simulink model "AMCLIB_FWSpeedLoop_BAM_F16"  (Simulink 8.3)
settings: Solver=ode45  StartTime=0.0  StopTime=10.0  RelTol=1e-3
undefined symbols (not defined in the file): f16IntegGainFW, f16IntegGainQ, f16PropGainFW, f16PropGainQ, f32RampDown, f32RampUp, s16IntegGainShiftFW, s16IntegGainShiftQ, s16PropGainShiftFW, s16PropGainShiftQ, u16NSamplesFW, u16NSamplesW
settings Model: Creator=nxa18952  LastModifiedBy=nxa18952
settings DataIOCC: SignalLoggingSaveFormat=Dataset
settings DebuggingCC: UnderspecifiedInitializationDetection=Simplified  StateNameClashWarn=none
settings GRTTargetCC: CombineOutputUpdateFcns=on  GRTInterface=off

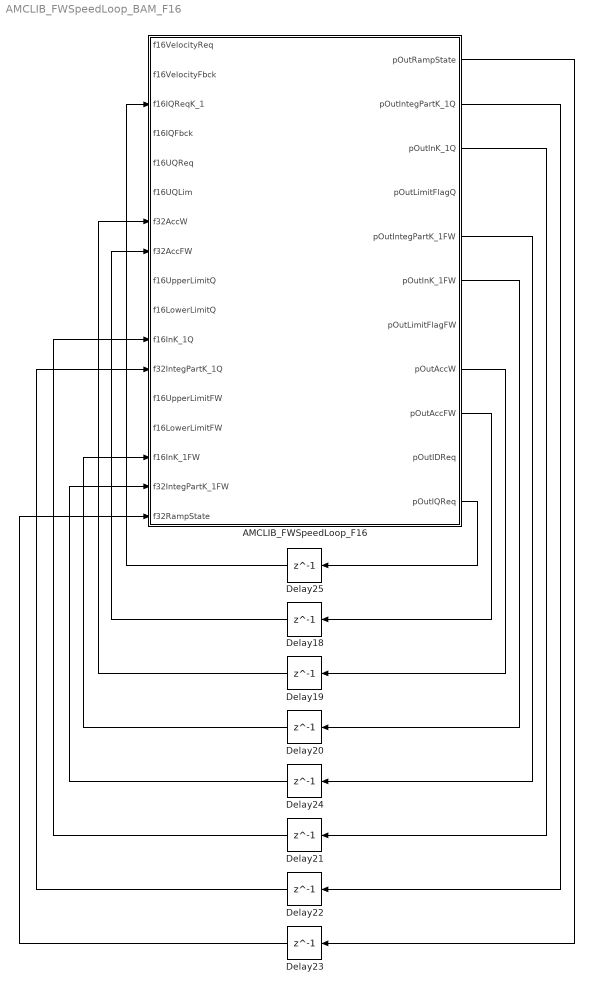
== system AMCLIB_FWSpeedLoop_BAM_F16 ==
  AMCLIB_FWSpeedLoop_F16 : Subsystem  mask(AMCLIB_FWSpeedLoop_F16){u16NSamplesW=u16NSamplesW, u16NSamplesFW=u16NSamplesFW, f16PropGainQ=f16PropGainQ, s16PropGainShiftQ=s16PropGainShiftQ, f16IntegGainQ=f16IntegGainQ, s16IntegGainShiftQ=s16IntegGainShiftQ, f16PropGainFW=f16PropGainFW, s16PropGainShiftFW=s16PropGainShiftFW, f16IntegGainFW=f16IntegGainFW, s16IntegGainShiftFW=s16IntegGainShiftFW, f32RampUp=f32RampUp, f32RampDown=f32RampDown}
      mask help: Bit accurate model of the speed loop algorithm with field weakening capability in 16-bit fixed-point implementation.
      mask init:
      | pos = get_param(gcb, 'Position');width = pos(3) - pos(1); height = pos(4) - pos(2);tX=width/2;tY=height*0.9;
      mask Display: color('black');port_label('input',1,'f16VelocityReq');port_label('input',2,'f16VelocityFbck');port_label('input',3,'f16IQReqK_1');port_label('input',4,'f16IQFbck');port_label('input',5,'f16UQReq');port_label('input',6,'f16UQLim');port_label('input',7,'f32AccW');port_label('input',8,'f32AccFW');port_label('input',9,'f16UpperLimitQ');port_label('input',10,'f16LowerLimitQ');port_label('input',11,'f16InK_1Q');port_label('input',12,'f32IntegPartK_1Q');port_label('input',13,'f16UpperLimitFW');port_label('input',14,'f16LowerLimitFW');port_label('input',15,'f16InK_1FW');port_label('input',16,'f32IntegPartK_1FW');port_label('input',17,'f32RampState');port_label('output',1,'pOutRampState');port_label('output',2,'pOutIntegPartK_1Q');port_label('output',3,'pOutInK_1Q');port_label('output',4,'pOutLimitFlagQ');port_label('output',5,'pOutIntegPartK_1FW');port_label('output',6,'pOutInK_1FW');port_label('output',7,'pOutLimitFlagFW');port_label('output',8,'pOutAccW');port_label('output',9,'pOutAccFW');port_label('output',10,'pOutIDReq');port_label('output',11,'pOutIQReq');color('black');disp('AMCLIB_FWSpeedLoop_F16');color('blue');text(tX,tY, 'BAM', 'horizontalAlignment', 'center');
  Delay{18..25} (8 alike) : Delay  DelayLength=1  InitialCondition=0
  wires:
  AMCLIB_FWSpeedLoop_F16/11(pOutIQReq) -> Delay25/1
  AMCLIB_FWSpeedLoop_F16/9(pOutAccFW) -> Delay18/1
  AMCLIB_FWSpeedLoop_F16/8(pOutAccW) -> Delay19/1
  AMCLIB_FWSpeedLoop_F16/6(pOutInK_1FW) -> Delay20/1
  AMCLIB_FWSpeedLoop_F16/5(pOutIntegPartK_1FW) -> Delay24/1
  AMCLIB_FWSpeedLoop_F16/3(pOutInK_1Q) -> Delay21/1
  AMCLIB_FWSpeedLoop_F16/2(pOutIntegPartK_1Q) -> Delay22/1
  AMCLIB_FWSpeedLoop_F16/1(pOutRampState) -> Delay23/1
  Delay25/1 -> AMCLIB_FWSpeedLoop_F16/3(f16IQReqK_1)
  Delay18/1 -> AMCLIB_FWSpeedLoop_F16/8(f32AccFW)
  Delay19/1 -> AMCLIB_FWSpeedLoop_F16/7(f32AccW)
  Delay20/1 -> AMCLIB_FWSpeedLoop_F16/15(f16InK_1FW)
  Delay24/1 -> AMCLIB_FWSpeedLoop_F16/16(f32IntegPartK_1FW)
  Delay21/1 -> AMCLIB_FWSpeedLoop_F16/11(f16InK_1Q)
  Delay22/1 -> AMCLIB_FWSpeedLoop_F16/12(f32IntegPartK_1Q)
  Delay23/1 -> AMCLIB_FWSpeedLoop_F16/17(f32RampState)

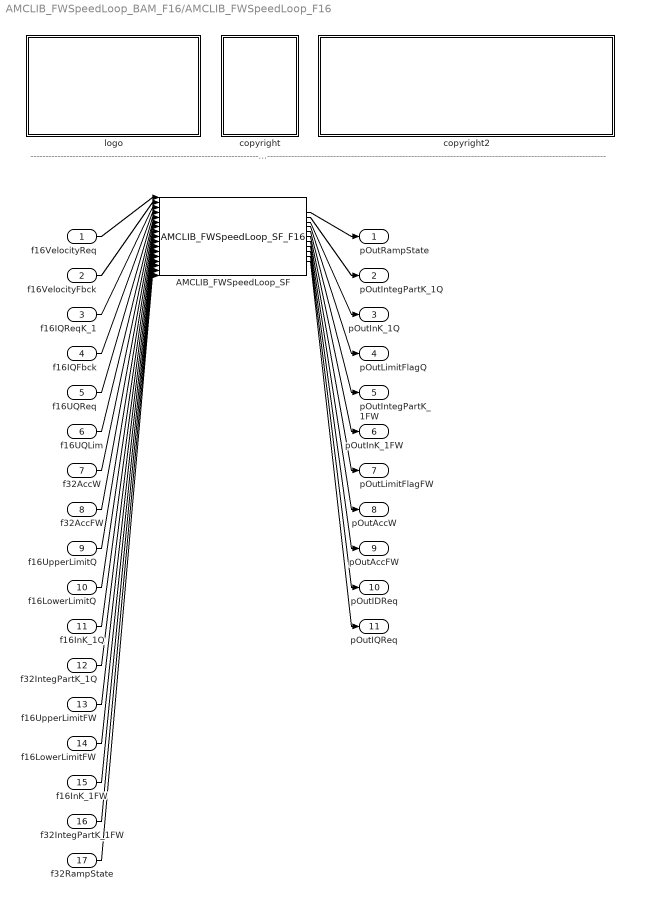
== system AMCLIB_FWSpeedLoop_BAM_F16/AMCLIB_FWSpeedLoop_F16 ==
  note: ---------------------------------------------------------------------------------------------------------------------------------------------------------------------------------------------------
  f16VelocityReq : Inport
  f16VelocityFbck : Inport  Port=2
  f16IQReqK_1 : Inport  Port=3
  f16IQFbck : Inport  Port=4
  f16UQReq : Inport  Port=5
  f16UQLim : Inport  Port=6
  f32AccW : Inport  Port=7
  f32AccFW : Inport  Port=8
  f16UpperLimitQ : Inport  Port=9
  f16LowerLimitQ : Inport  Port=10
  f16InK_1Q : Inport  Port=11
  f32IntegPartK_1Q : Inport  Port=12
  f16UpperLimitFW : Inport  Port=13
  f16LowerLimitFW : Inport  Port=14
  f16InK_1FW : Inport  Port=15
  f32IntegPartK_1FW : Inport  Port=16
  f32RampState : Inport  Port=17
  AMCLIB_FWSpeedLoop_SF : S-Function  FunctionName=AMCLIB_FWSpeedLoop_SF_F16  Parameters=u16NSamplesW,u16NSamplesFW,f16PropGainQ,s16PropGainShiftQ,f16IntegGainQ,s16IntegGainShiftQ,f16PropGainFW,s16PropGainShiftFW,f16IntegGainFW,s16IntegGainShiftFW,f32RampUp,f32RampDown  EnableBusSupport=off
  copyright : Subsystem
      mask Display: text(10,90,'FILE:');text(10,75,'DESRIPTION:');text(10,60,'COPYRIGHT:');text(10,45,'VERSION:');text(10,30,'DATE:')
  copyright2 : Subsystem
      mask Display: text(10,90,'AMCLIB_FWSpeedLoop_BAM_F16.mdl');text(10,75,'Speed Loop with Field Weakening.');text(10,60,'NXP');text(10,45,'1.0');text(10,30,'17-Apr-2018');
  logo : Subsystem
      mask Display: image(imread('logo.jpg'))
  pOutRampState : Outport
  pOutIntegPartK_1Q : Outport  Port=2
  pOutInK_1Q : Outport  Port=3
  pOutLimitFlagQ : Outport  Port=4
  pOutIntegPartK_1FW : Outport  Port=5
  pOutInK_1FW : Outport  Port=6
  pOutLimitFlagFW : Outport  Port=7
  pOutAccW : Outport  Port=8
  pOutAccFW : Outport  Port=9
  pOutIDReq : Outport  Port=10
  pOutIQReq : Outport  Port=11
  wires:
  f16VelocityReq/1 -> AMCLIB_FWSpeedLoop_SF/1
  f16VelocityFbck/1 -> AMCLIB_FWSpeedLoop_SF/2
  f16IQReqK_1/1 -> AMCLIB_FWSpeedLoop_SF/3
  f16IQFbck/1 -> AMCLIB_FWSpeedLoop_SF/4
  f16UQReq/1 -> AMCLIB_FWSpeedLoop_SF/5
  f16UQLim/1 -> AMCLIB_FWSpeedLoop_SF/6
  f32AccW/1 -> AMCLIB_FWSpeedLoop_SF/7
  f32AccFW/1 -> AMCLIB_FWSpeedLoop_SF/8
  f16UpperLimitQ/1 -> AMCLIB_FWSpeedLoop_SF/9
  f16LowerLimitQ/1 -> AMCLIB_FWSpeedLoop_SF/10
  f16InK_1Q/1 -> AMCLIB_FWSpeedLoop_SF/11
  f32IntegPartK_1Q/1 -> AMCLIB_FWSpeedLoop_SF/12
  f16UpperLimitFW/1 -> AMCLIB_FWSpeedLoop_SF/13
  f16LowerLimitFW/1 -> AMCLIB_FWSpeedLoop_SF/14
  f16InK_1FW/1 -> AMCLIB_FWSpeedLoop_SF/15
  f32IntegPartK_1FW/1 -> AMCLIB_FWSpeedLoop_SF/16
  f32RampState/1 -> AMCLIB_FWSpeedLoop_SF/17
  AMCLIB_FWSpeedLoop_SF/1 -> pOutRampState/1
  AMCLIB_FWSpeedLoop_SF/2 -> pOutIntegPartK_1Q/1
  AMCLIB_FWSpeedLoop_SF/3 -> pOutInK_1Q/1
  AMCLIB_FWSpeedLoop_SF/4 -> pOutLimitFlagQ/1
  AMCLIB_FWSpeedLoop_SF/5 -> pOutIntegPartK_1FW/1
  AMCLIB_FWSpeedLoop_SF/6 -> pOutInK_1FW/1
  AMCLIB_FWSpeedLoop_SF/7 -> pOutLimitFlagFW/1
  AMCLIB_FWSpeedLoop_SF/8 -> pOutAccW/1
  AMCLIB_FWSpeedLoop_SF/9 -> pOutAccFW/1
  AMCLIB_FWSpeedLoop_SF/10 -> pOutIDReq/1
  AMCLIB_FWSpeedLoop_SF/11 -> pOutIQReq/1

== system AMCLIB_FWSpeedLoop_BAM_F16/AMCLIB_FWSpeedLoop_F16/copyright ==

== system AMCLIB_FWSpeedLoop_BAM_F16/AMCLIB_FWSpeedLoop_F16/copyright2 ==

== system AMCLIB_FWSpeedLoop_BAM_F16/AMCLIB_FWSpeedLoop_F16/logo ==
